simulink model "assignment_5"  (R2020b)
settings: Solver=VariableStepAuto  StartTime=0.0  StopTime=10.0  RelTol=1e-3
undefined symbols (not defined in the file): C, R
settings Model: Creator=Sudhanshu  LastModifiedBy=Sudhanshu

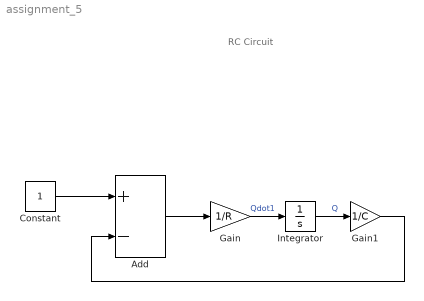
== system assignment_5 ==
  note: RC Circuit
  Add : Sum  Inputs=+-
  Constant : Constant
  Gain : Gain  Gain=1/R
  Gain1 : Gain  Gain=1/C
  Integrator : Integrator
  wires:
  Add/1 -> Gain/1
  Gain/1 -> Integrator/1  "Qdot1"
  Integrator/1 -> Gain1/1  "Q"
  Gain1/1 -> Add/2
  Constant/1 -> Add/1
